simulink model "Alarm_System_Simulink_Arduino"  (R2018a)
settings: Solver=VariableStepAuto  StartTime=0.0  StopTime=10.0  RelTol=1e-3
libraries: arduinolib x5
settings Model: Creator=Moataz  LastModifiedBy=Moataz

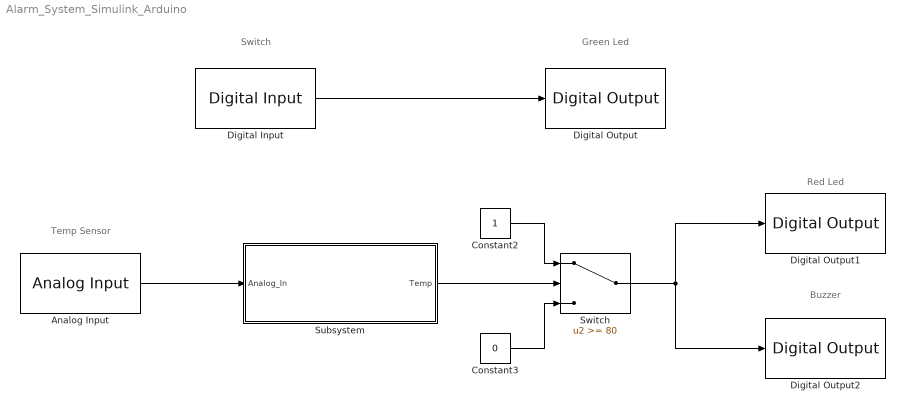
== system Alarm_System_Simulink_Arduino ==
  note: Buzzer
  note: Red Led
  note: Temp Sensor
  note: Green Led
  note: Switch
  Analog Input : arduinolib/Analog Input  pinNumber=4  ReadResultsOnly=off  ConversionTriggerSource=Software  ExternalTriggerType=uint32(0)  OutputDataType=uint16  EnableConversionCompleteNotify=off  EnableOuputStatus=off  SampleTime=1  blockPlatform=arduino
  Constant2 : Constant
  Constant3 : Constant  Value=0
  Digital Input : arduinolib/Digital Input  pinNumber=8  sampleTime=0.1  blockPlatform=arduino
      settings: SourceProductName=Simulink Support Package for Arduino Hardware
  Digital Output : arduinolib/Digital Output  pinNumber=9  blockPlatform=arduino
  Digital Output1 : arduinolib/Digital Output  pinNumber=9  blockPlatform=arduino
  Digital Output2 : arduinolib/Digital Output  pinNumber=9  blockPlatform=arduino
  Subsystem : Subsystem
  Switch : Switch  Threshold=80
  wires:
  Digital Input/1 -> Digital Output/1
  Analog Input/1 -> Subsystem/1(Analog_In)
  Constant3/1 -> Switch/3
  Constant2/1 -> Switch/1
  Subsystem/1(Temp) -> Switch/2
  Switch/1 -> Digital Output1/1, Digital Output2/1

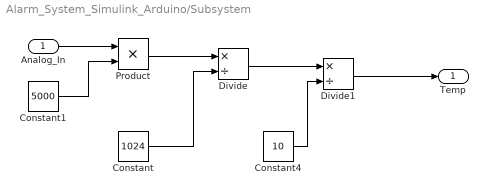
== system Alarm_System_Simulink_Arduino/Subsystem ==
  Analog_In : Inport
  Constant : Constant  Value=1024
  Constant1 : Constant  Value=5000
  Constant4 : Constant  Value=10
  Divide : Product  Inputs=*/
  Divide1 : Product  Inputs=*/
  Product : Product
  Temp : Outport
  wires:
  Constant/1 -> Divide/2
  Constant1/1 -> Product/2
  Analog_In/1 -> Product/1
  Product/1 -> Divide/1
  Divide/1 -> Divide1/1
  Constant4/1 -> Divide1/2
  Divide1/1 -> Temp/1
